simulink model "IV_2018B_error_test"  (R2018b)
settings: Solver=VariableStepAuto  StartTime=0.0  StopTime=10.0  RelTol=1e-3
libraries: fl_lib x17, nesl_utility x10
settings Model: Creator=94840  LastModifiedBy=yangr

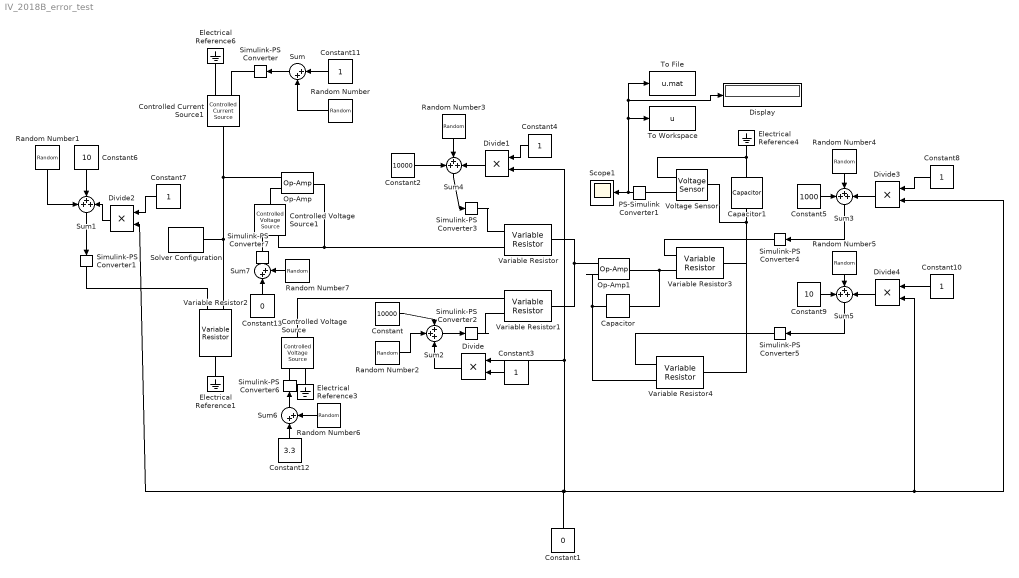
== system IV_2018B_error_test ==
  Capacitor : fl_lib/Electrical/Electrical Elements/Capacitor  c=10e-6 F  r=1e-6 Ohm  g=0 1/Ohm  i_specify=off  i_priority=None  i=0 A  i_nominal_specify=off  i_nominal_unit=A  i_nominal_value=1  v_specify=off  v_priority=None  v=0 V  v_nominal_specify=off  v_nominal_unit=V  v_nominal_value=1  vc_specify=off  vc_priority=High  vc=0 V  vc_nominal_specify=off  vc_nominal_unit=V  vc_nominal_value=1
  Capacitor1 : fl_lib/Electrical/Electrical Elements/Capacitor  c=10e-12 F  r=1e-6 Ohm  g=0 1/Ohm  i_specify=off  i_priority=None  i=0 A  i_nominal_specify=off  i_nominal_unit=A  i_nominal_value=1  v_specify=off  v_priority=None  v=0 V  v_nominal_specify=off  v_nominal_unit=V  v_nominal_value=1  vc_specify=off  vc_priority=High  vc=0 V  vc_nominal_specify=off  vc_nominal_unit=V  vc_nominal_value=1
  Constant : Constant  Value=10000
  Constant1 : Constant  Value=0
  Constant{3..4,7..8,10..11} (6 alike) : Constant
  Constant12 : Constant  Value=3.3
  Constant13 : Constant  Value=0
  Constant2 : Constant  Value=10000
  Constant5 : Constant  Value=1000
  Constant6 : Constant  Value=10
  Constant9 : Constant  Value=10
  Controlled Current Source1 : fl_lib/Electrical/Electrical Sources/Controlled Current Source
  Controlled Voltage Source : fl_lib/Electrical/Electrical Sources/Controlled Voltage Source
  Controlled Voltage Source1 : fl_lib/Electrical/Electrical Sources/Controlled Voltage Source
  Display : Display
  Divide{,1..4} (5 alike) : Product  Inputs=**
  Electrical Reference{1,3..4,6} (4 alike) : fl_lib/Electrical/Electrical Elements/Electrical Reference
  Op-Amp : fl_lib/Electrical/Electrical Elements/Op-Amp  outI_specify=off  outI_priority=None  outI=0 A  outI_nominal_specify=off  outI_nominal_unit=A  outI_nominal_value=1
  Op-Amp1 : fl_lib/Electrical/Electrical Elements/Op-Amp  outI_specify=off  outI_priority=None  outI=0 A  outI_nominal_specify=off  outI_nominal_unit=A  outI_nominal_value=1
  PS-Simulink Converter1 : nesl_utility/PS-Simulink Converter  PhysicalDomain=network_engine_domain  SubClassName=ps_output  LeftPortType=input  RightPortType=output  PseudoPeriodic=off  Frequencies=[]  Unit=1  AffineConversion=off
  Random Number : RandomNumber  Variance=0  SampleTime=0.1
  Random Number1 : RandomNumber  Variance=0  SampleTime=0.001
  Random Number2 : RandomNumber  Variance=0  Seed=3  SampleTime=0.001
  Random Number3 : RandomNumber  Variance=0  SampleTime=0.001
  Random Number4 : RandomNumber  Variance=1000  SampleTime=0.001
  Random Number5 : RandomNumber  Variance=10  SampleTime=0.001
  Random Number6 : RandomNumber  Variance=0  SampleTime=0.1
  Random Number7 : RandomNumber  Variance=0  SampleTime=0.01
  Scope1 : Scope
  Simulink-PS Converter{,1..7} (8 alike) : nesl_utility/Simulink-PS Converter  PhysicalDomain=network_engine_domain  SubClassName=ps_input  LeftPortType=input  RightPortType=output  PseudoPeriodic=off  Frequencies=[]  NoiseDistribution=none  NoiseParameters=[]  Unit=1  AffineConversion=off  FilteringAndDerivatives=provide  SimscapeFilterOrder=1  InputFilterTimeConstant=0.001  UdotUserProvided=0
  Solver Configuration : nesl_utility/Solver Configuration  PhysicalDomain=network_engine_domain  SubClassName=solver  LeftPortType=input  RightPortType=generic  Tones=[]  Harmonics=[]  SimulateNoise=off  Profile=off  UseLocalSampling=off  EnableSwitchedLinearOptims=on  FrequencyDomain=off  UseCCode=off  RelTol=0.001  AbsTol=1e-06  MinStep=1e-09  ToWorkspace=off  RevertToSquareIcSolve=off  NumHomotopyIterations=100  PhasorMode=off  PhasorModeNumHarmonics=1  DoDC=off  ResidualTolerance=1e-09  UseLocalSolver=off  LocalSolverChoice=NE_BACKWARD_EULER_ADVANCER  LocalSolverSampleTime=0.001  DoFixedCost=off  MaxNonlinIter=3  MaxModeIter=2  LinearAlgebra=auto  EquationFormulation=NE_TIME_EF  DelaysMemoryBudget=1024  AutomaticFiltering=on  FilteringTimeConstant=0.001  PartitionStorageMethod=AS_NEEDED  PartitionMemoryBudget=1024
  Sum : Sum  Inputs=|++
  Sum{1..5} (5 alike) : Sum  Inputs=+++
  Sum6 : Sum  Inputs=|++
  Sum7 : Sum  Inputs=|++
  To File : ToFile  Filename=u.mat
  To Workspace : ToWorkspace  VariableName=u  SampleTime=-1
      settings: Save2DSignal=2-D array (concatenate along first dimension)
  Variable Resistor{,1..4} (5 alike) : fl_lib/Electrical/Electrical Elements/Variable Resistor  Rmin=0 Ohm  i_specify=off  i_priority=None  i=0 A  i_nominal_specify=off  i_nominal_unit=A  i_nominal_value=1  v_specify=off  v_priority=None  v=0 V  v_nominal_specify=off  v_nominal_unit=V  v_nominal_value=1
  Voltage Sensor : fl_lib/Electrical/Electrical Sensors/Voltage Sensor
  wires:
  Sum1/1 -> Simulink-PS Converter1/1
  Sum2/1 -> Simulink-PS Converter2/1
  Random Number2/1 -> Sum2/2
  Constant/1 -> Sum2/1
  PS-Simulink Converter1/1 -> Display/1, To File/1, To Workspace/1, Scope1/1
  Random Number1/1 -> Sum1/1
  Random Number3/1 -> Sum4/2
  Constant1/1 -> Divide3/2, Divide4/2, Divide/1, Divide1/2, Divide2/2
  Divide/1 -> Sum2/3
  Sum4/1 -> Simulink-PS Converter3/1
  Constant2/1 -> Sum4/1
  Divide1/1 -> Sum4/3
  Constant3/1 -> Divide/2
  Constant4/1 -> Divide1/1
  Constant6/1 -> Sum1/2
  Divide2/1 -> Sum1/3
  Constant7/1 -> Divide2/1
  Constant5/1 -> Sum3/1
  Constant8/1 -> Divide3/1
  Divide3/1 -> Sum3/3
  Random Number4/1 -> Sum3/2
  Sum3/1 -> Simulink-PS Converter4/1
  Random Number5/1 -> Sum5/2
  Divide4/1 -> Sum5/3
  Sum5/1 -> Simulink-PS Converter5/1
  Constant9/1 -> Sum5/1
  Constant10/1 -> Divide4/1
  Random Number/1 -> Sum/2
  Sum/1 -> Simulink-PS Converter/1
  Constant11/1 -> Sum/1
  Sum6/1 -> Simulink-PS Converter6/1
  Constant12/1 -> Sum6/1
  Random Number6/1 -> Sum6/2
  Random Number7/1 -> Sum7/2
  Constant13/1 -> Sum7/1
  Sum7/1 -> Simulink-PS Converter7/1
  connections:
  Op-Amp/LConn1 -- Solver Configuration/RConn1 -- Variable Resistor2/LConn2 -- Controlled Current Source1/LConn1
  Simulink-PS Converter1/RConn1 -- Variable Resistor2/LConn1
  Simulink-PS Converter2/RConn1 -- Variable Resistor1/LConn1
  Simulink-PS Converter3/RConn1 -- Variable Resistor/LConn1
  Electrical Reference1/LConn1 -- Variable Resistor2/RConn1
  Variable Resistor1/LConn2 -- Controlled Voltage Source/LConn1
  Electrical Reference3/LConn1 -- Controlled Voltage Source/RConn2
  Variable Resistor/RConn1 -- Op-Amp1/LConn1 -- Variable Resistor1/RConn1
  Variable Resistor3/LConn2 -- Op-Amp1/RConn1 -- Capacitor/RConn1
  Op-Amp1/LConn2 -- Variable Resistor4/LConn2 -- Capacitor/LConn1
  Voltage Sensor/LConn1 -- Variable Resistor4/RConn1 -- Variable Resistor3/RConn1 -- Capacitor1/LConn1
  Electrical Reference4/LConn1 -- Voltage Sensor/RConn2 -- Capacitor1/RConn1
  PS-Simulink Converter1/LConn1 -- Voltage Sensor/RConn1
  Simulink-PS Converter4/RConn1 -- Variable Resistor3/LConn1
  Simulink-PS Converter5/RConn1 -- Variable Resistor4/LConn1
  Simulink-PS Converter/RConn1 -- Controlled Current Source1/RConn1
  Electrical Reference6/LConn1 -- Controlled Current Source1/RConn2
  Op-Amp/RConn1 -- Controlled Voltage Source1/RConn2 -- Variable Resistor/LConn2
  Simulink-PS Converter6/RConn1 -- Controlled Voltage Source/RConn1
  Op-Amp/LConn2 -- Controlled Voltage Source1/LConn1
  Simulink-PS Converter7/RConn1 -- Controlled Voltage Source1/RConn1
